simulink model "Problem2"  (R2020a)
settings: Solver=VariableStepAuto  StartTime=0.0  StopTime=100  RelTol=1e-3
undefined symbols (not defined in the file): b1, k1, k2, m1, m2
settings Model: Creator=sreeram  LastModifiedBy=sreeram
settings DataIOCC: ExternalInput=[t, stin]  LoadExternalInput=on

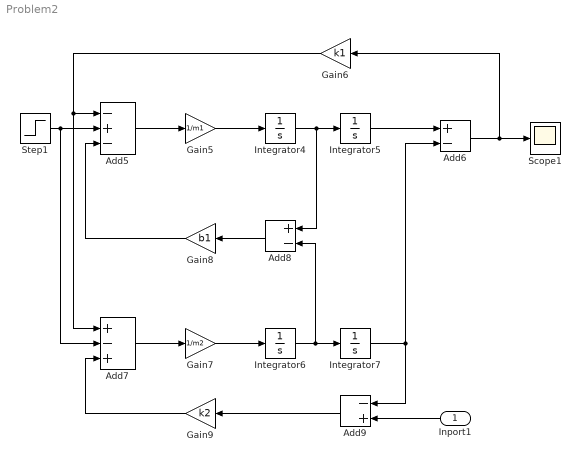
== system Problem2 ==
  Inport1 : Inport
  Add5 : Sum  Inputs=-+-
  Add6 : Sum  Inputs=+-
  Add7 : Sum  Inputs=+-+
  Add8 : Sum  Inputs=+-
  Add9 : Sum  Inputs=-+
  Gain5 : Gain  Gain=1/m1
  Gain6 : Gain  Gain=k1
  Gain7 : Gain  Gain=1/m2
  Gain8 : Gain  Gain=b1
  Gain9 : Gain  Gain=k2
  Integrator{4..7} (4 alike) : Integrator
  Scope1 : Scope
  Step1 : Step  SampleTime=0
  wires:
  Step1/1 -> Add7/2, Add5/2
  Add5/1 -> Gain5/1
  Gain5/1 -> Integrator4/1
  Integrator4/1 -> Add8/1, Integrator5/1
  Integrator5/1 -> Add6/1
  Add6/1 -> Gain6/1, Scope1/1
  Gain6/1 -> Add7/1, Add5/1
  Add7/1 -> Gain7/1
  Gain7/1 -> Integrator6/1
  Integrator6/1 -> Add8/2, Integrator7/1
  Integrator7/1 -> Add9/1, Add6/2
  Add8/1 -> Gain8/1
  Gain8/1 -> Add5/3
  Inport1/1 -> Add9/2
  Add9/1 -> Gain9/1
  Gain9/1 -> Add7/3
